simulink model "Laurenz_Simulink"  (R2020a)
settings: Solver=VariableStepAuto  StartTime=0.0  StopTime=250  RelTol=1e-3
settings Model: Creator=User  LastModifiedBy=User

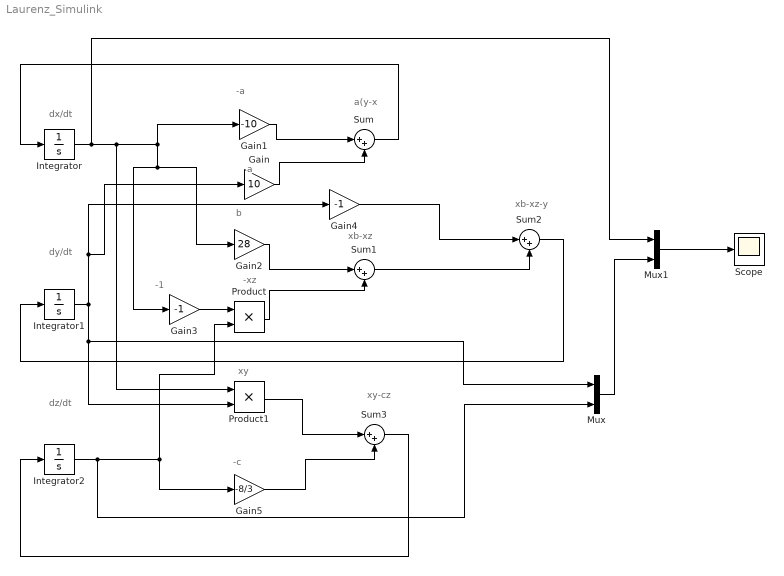
== system Laurenz_Simulink ==
  note: xy-cz
  note: -c
  note: xy
  note: xb-xz-y
  note: xb-xz
  note: -xz
  note: -1
  note: b
  note: a(y-x
  note: a
  note: -a
  note: dx/dt
  note: dy/dt
  note: dz/dt
  Gain : Gain  Gain=10
  Gain1 : Gain  Gain=-10
  Gain2 : Gain  Gain=28
  Gain3 : Gain  Gain=-1
  Gain4 : Gain  Gain=-1
  Gain5 : Gain  Gain=-8/3
  Integrator : Integrator  InitialCondition=2.01
  Integrator1 : Integrator  InitialCondition=3.1
  Integrator2 : Integrator  InitialCondition=8.2
  Mux : Mux  Inputs=2
  Mux1 : Mux  Inputs=2
  Product : Product
  Product1 : Product
  Scope : Scope
  Sum{,1..3} (4 alike) : Sum  Inputs=|++
  wires:
  Integrator1/1 -> Product1/2, Mux/1, Gain4/1, Gain/1
  Integrator/1 -> Mux1/1, Gain3/1, Gain2/1, Gain1/1, Product1/1
  Gain/1 -> Sum/2
  Gain1/1 -> Sum/1
  Gain3/1 -> Product/1
  Integrator2/1 -> Mux/2, Gain5/1, Product/2
  Product/1 -> Sum1/2
  Gain2/1 -> Sum1/1
  Sum1/1 -> Sum2/2
  Gain4/1 -> Sum2/1
  Gain5/1 -> Sum3/2
  Product1/1 -> Sum3/1
  Sum3/1 -> Integrator2/1
  Sum2/1 -> Integrator1/1
  Sum/1 -> Integrator/1
  Mux/1 -> Mux1/2
  Mux1/1 -> Scope/1
